simulink model "fuzzu_commande"  (R2022b)
settings: Solver=VariableStepAuto  StartTime=0.0  StopTime=100  RelTol=1e-3
values from neighbouring files (symbols this model uses):
  Ao = [-1/60, 0; 0, -1/30]    [tp.m]
  Bo = [1, 0; -0.05, 0.05]    [tp.m]
  Co = eye(2)    [tp.m]
  Do = zeros(2)    [tp.m]
  Te = 6    [fuzzy_cuve.m]    (also in tp.m)
libraries: fuzblock x1
settings Model: Creator=lyeromona522  LastModifiedBy=lyeromona522

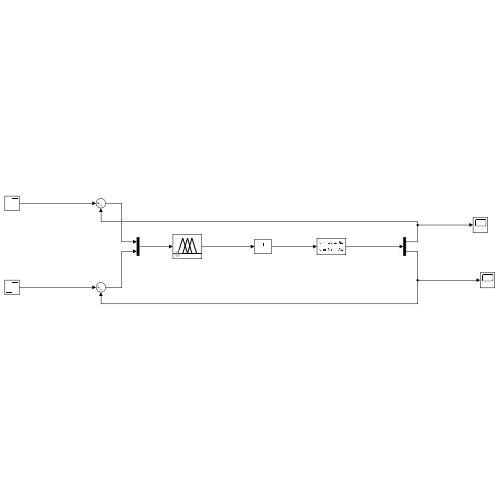
[thumbnail: Simulink's stored preview of the top-level diagram]
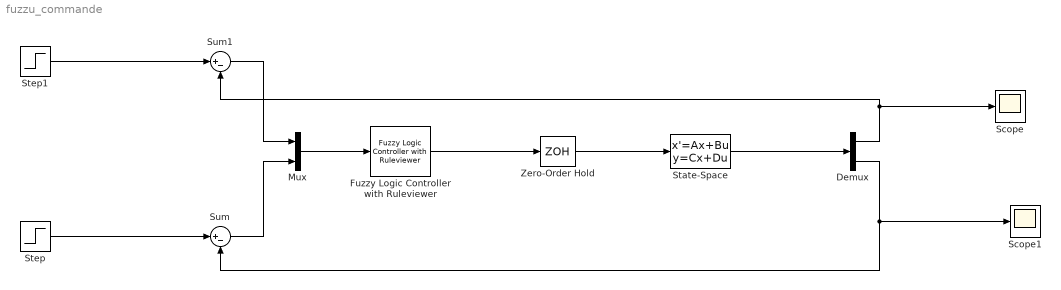
== system fuzzu_commande ==
  Demux : Demux  Outputs=2
  Fuzzy Logic Controller with Ruleviewer : fuzblock/Fuzzy Logic  Controller  with Ruleviewer  fismatrix=fuzzy_cuve  Ts=2
  Mux : Mux  Inputs=2
  Scope : Scope
  Scope1 : Scope
  State-Space : StateSpace  A=Ao  B=Bo  C=Co  D=Do  InitialCondition=0
  Step : Step  SampleTime=0
  Step1 : Step  After=50  SampleTime=0
  Sum : Sum  Inputs=|+-
  Sum1 : Sum  Inputs=|+-
  Zero-Order Hold : ZeroOrderHold  SampleTime=Te
  wires:
  Step/1 -> Sum/1
  Step1/1 -> Sum1/1
  Sum1/1 -> Mux/1
  Sum/1 -> Mux/2
  Mux/1 -> Fuzzy Logic Controller with Ruleviewer/1
  Fuzzy Logic Controller with Ruleviewer/1 -> Zero-Order Hold/1
  Zero-Order Hold/1 -> State-Space/1
  State-Space/1 -> Demux/1
  Demux/2 -> Scope1/1, Sum/2
  Demux/1 -> Scope/1, Sum1/2
